simulink model "yoyo_sim_noFSM"  (R2013b)
settings: Solver=ode45  StartTime=0.0  StopTime=10.0  RelTol=1e-3
values from neighbouring files (symbols this model uses):
  downA = [0,1;0,-r*epsilon/(I+m*r^2)]    [yoyo_model_simulate.m]
  downB = [0;m*r/(I+m*r^2)]    [yoyo_model_simulate.m]
  newC = [1,1]    [yoyo_model_simulate.m]
  PARAMS = struct(f1,v1,f2,v2,f3,v3,f4,v4,f5,v5,f6,v6,f7,v7,f8,v8,f9,v9,f10,v10,f11,v11,f12,v12,f13,v13)    [yoyo_model.m]    (also in yoyo_model_simulate.m = struct(f1,v1,f2,v2,f3,v3,f4,v4,f5,v5,f6,v6,f7,v7,f8,v8,f9,v9; yoyo_model_testing_lqi.m)
  upB = [0;-m*r/(I+m*r^2)]    [yoyo_model_simulate.m]
settings Model: Creator=thomasesch  LastModifiedBy=thomasesch

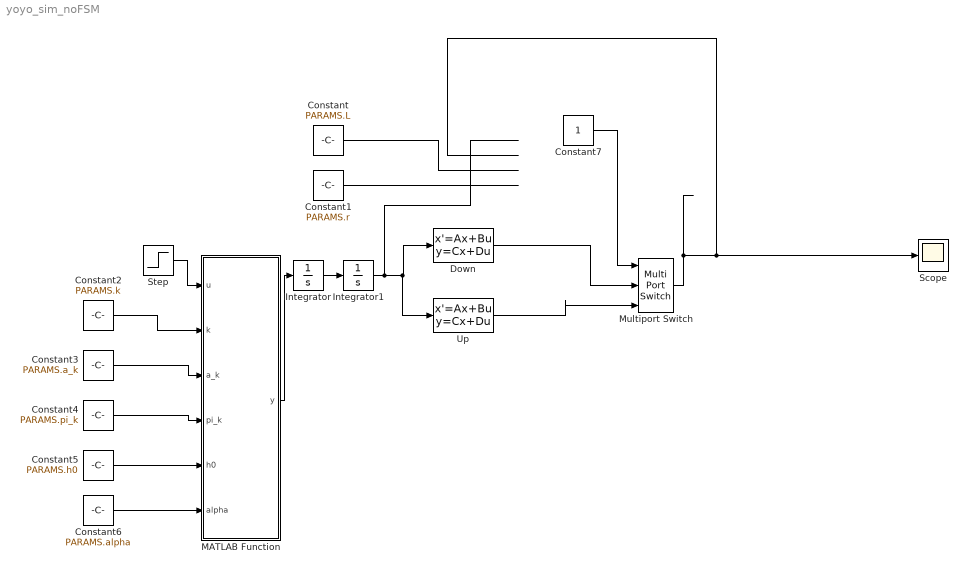
== system yoyo_sim_noFSM ==
  Constant : Constant  Value=PARAMS.L
  Constant1 : Constant  Value=PARAMS.r
  Constant2 : Constant  Value=PARAMS.k
  Constant3 : Constant  Value=PARAMS.a_k
  Constant4 : Constant  Value=PARAMS.pi_k
  Constant5 : Constant  Value=PARAMS.h0
  Constant6 : Constant  Value=PARAMS.alpha
  Constant7 : Constant
  Down : StateSpace  A=downA  B=downB  C=newC  D=0  X0=0
  Integrator : Integrator
  Integrator1 : Integrator
  MATLAB Function : MATLAB Function  TreatAsAtomicUnit=on
  Multiport Switch : MultiPortSwitch  Inputs=2
  Scope : Scope
  Step : Step  SampleTime=0
  Up : StateSpace  A=downA  B=upB  C=newC  D=0  X0=0
  wires:
  Up/1 -> Multiport Switch/3
  Down/1 -> Multiport Switch/2
  Integrator/1 -> Integrator1/1
  Integrator1/1 -> Up/1, Down/1
  Constant1/1 -> ?
  Constant/1 -> ?
  Multiport Switch/1 -> Scope/1
  MATLAB Function/1(y) -> Integrator/1
  Step/1 -> MATLAB Function/1(u)
  Constant2/1 -> MATLAB Function/2(k)
  Constant3/1 -> MATLAB Function/3(a_k)
  Constant4/1 -> MATLAB Function/4(pi_k)
  Constant5/1 -> MATLAB Function/5(h0)
  Constant6/1 -> MATLAB Function/6(alpha)
  Constant7/1 -> Multiport Switch/1

== matlab function yoyo_sim_noFSM/MATLAB Function ==
  data: u input; y output; k input; a_k input; pi_k input; h0 input; alpha input
function y = fcn(u,k,a_k,pi_k,h0,alpha)
%#codegen


hot = 0;
for k = 1:k
    hot = hot + a_k(k)*sin(pi_k(k)*u);
end
hot = h0 + alpha*hot;


y = hot;
